simulink model "mcp3202_task"  (Simulink 3.00)
libraries: mathlib x3, speclib x1, arclib x1

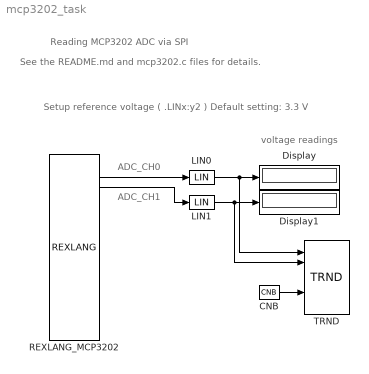
== system mcp3202_task ==
  note: See the README.md and mcp3202.c files for details.
  note: Reading MCP3202 ADC via SPI
  note: voltage readings
  note: ADC_CH0
  note: ADC_CH1
  note: Setup reference voltage ( .LINx:y2 )
      | Default setting: 3.3 V
  CNB : mathlib/CNB  YCN=on
  Display : Display
      settings: Format=short  Suffix=V
  Display1 : Display
      settings: Format=short  Suffix=V
  LIN0 : mathlib/LIN  u1=0  y1=0  u2=4095  y2=3.3
  LIN1 : mathlib/LIN  u1=0  y1=0  u2=4095  y2=3.3
  REXLANG_MCP3202 : speclib/REXLANG  strs=0  srcname=mcp3202.c  srctype=1: C-like  stack=0  debug=1: No check  fname=/dev/spidev0.0  p0=/dev/spidev0.0
  TRND : arclib/TRND  n=4  l=1000  btype=8: Double  ptype1=1: Store  ptype2=1: Store  ptype3=1: Store  ptype4=1: Store  pfac=1  afac=0  arc=0  id=1  Title=Channels 0..3  timesrc=1
  wires:
  CNB/1 -> TRND/5
  LIN0/1 -> Display/1, TRND/1
  LIN1/1 -> Display1/1, TRND/2
  REXLANG_MCP3202/2 -> LIN0/1
  REXLANG_MCP3202/3 -> LIN1/1
